simulink model "emulation"  (R2022b)
settings: Solver=FixedStepAuto  StartTime=0.0  StopTime=0.2  FixedStep=5e-8  RelTol=1e-3
libraries: spsVoltageMeasurementLib x5, fl_lib x4, spsParallelRLCBranchLib x4, spsACVoltageSourceLib x3, spsSecondOrderFilterLib x1, ee_lib x1, spspowerguiLib x1
settings Model: Creator=Motimon  LastModifiedBy=HP
settings ModelReferenceCC: EnableRefExpFcnMdlSchedulingChecks=on

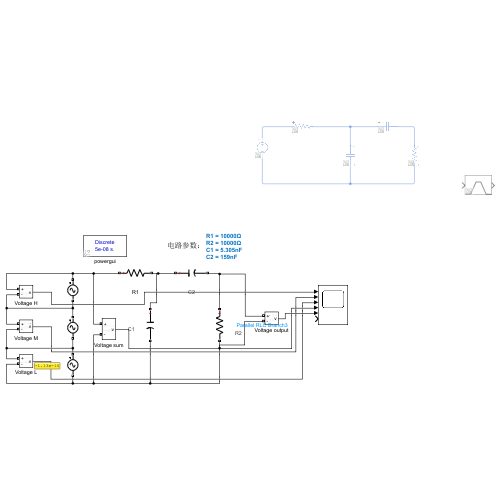
[thumbnail: Simulink's stored preview of the top-level diagram]
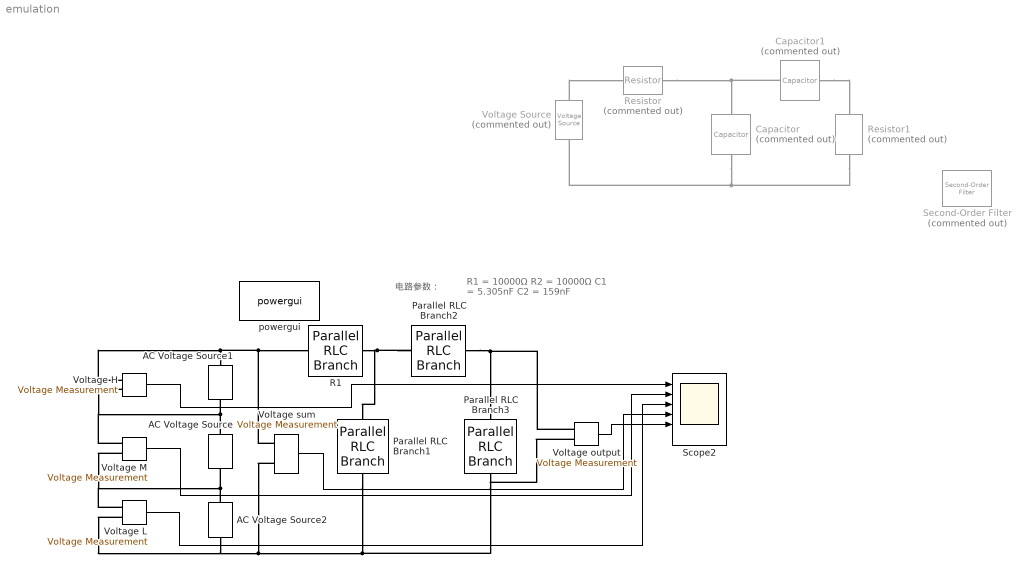
== system emulation ==
  note: 电路参数：
  note: R1 = 10000Ω
      | R2 = 10000Ω
      | C1 = 5.305nF
      | C2 = 159nF
  AC Voltage Source : spsACVoltageSourceLib/AC Voltage Source  Amplitude=0.5  Phase=0  Frequency=1550  SampleTime=0  Measurements=Voltage  BusType=swing  Pref=10e3  Qref=0  Qmin=-inf  Qmax=+inf
  AC Voltage Source1 : spsACVoltageSourceLib/AC Voltage Source  Amplitude=0.5  Phase=0  Frequency=60000  SampleTime=0  Measurements=Voltage  BusType=swing  Pref=10e3  Qref=0  Qmin=-inf  Qmax=+inf
  AC Voltage Source2 : spsACVoltageSourceLib/AC Voltage Source  Amplitude=0.5  Phase=0  Frequency=10  SampleTime=0  Measurements=Voltage  BusType=swing  Pref=10e3  Qref=0  Qmin=-inf  Qmax=+inf
  Capacitor : fl_lib/Electrical/Electrical Elements/Capacitor  Commented=on  c=1e-6 F  r=1e-6 Ohm  g=0 1/Ohm  i_specify=off  i_priority=None  i=0 A  i_nominal_specify=off  i_nominal_unit=A  i_nominal_value=1  v_specify=off  v_priority=None  v=0 V  v_nominal_specify=off  v_nominal_unit=V  v_nominal_value=1  vc_specify=off  vc_priority=High  vc=0 V  vc_nominal_specify=off  vc_nominal_unit=V  vc_nominal_value=1
  Capacitor1 : fl_lib/Electrical/Electrical Elements/Capacitor  Commented=on  c=1e-6 F  r=1e-6 Ohm  g=0 1/Ohm  i_specify=off  i_priority=None  i=0 A  i_nominal_specify=off  i_nominal_unit=A  i_nominal_value=1  v_specify=off  v_priority=None  v=0 V  v_nominal_specify=off  v_nominal_unit=V  v_nominal_value=1  vc_specify=off  vc_priority=High  vc=0 V  vc_nominal_specify=off  vc_nominal_unit=V  vc_nominal_value=1
  Parallel RLC Branch1 : spsParallelRLCBranchLib/Parallel RLC Branch  LConnTagsString=a  RConnTagsString=__new0  BranchType=C  Resistance=1  Inductance=1e-3  SetiL0=off  InitialCurrent=0  Capacitance=5.305e-9  Setx0=off  InitialVoltage=0  Measurements=None
      settings: AttributesFormatString=C1\n
  Parallel RLC Branch2 : spsParallelRLCBranchLib/Parallel RLC Branch  LConnTagsString=a  RConnTagsString=__new0  BranchType=C  Resistance=1  Inductance=1e-3  SetiL0=off  InitialCurrent=0  Capacitance=159e-9  Setx0=off  InitialVoltage=0  Measurements=None
      settings: AttributesFormatString=C2\n
  Parallel RLC Branch3 : spsParallelRLCBranchLib/Parallel RLC Branch  LConnTagsString=a  RConnTagsString=__new0  BranchType=R  Resistance=10000  Inductance=1e-3  SetiL0=off  InitialCurrent=0  Capacitance=1e-6  Setx0=off  InitialVoltage=0  Measurements=None
      settings: AttributesFormatString=R2\n
  R1 : spsParallelRLCBranchLib/Parallel RLC Branch  LConnTagsString=a  RConnTagsString=__new0  BranchType=R  Resistance=10000  Inductance=1e-3  SetiL0=off  InitialCurrent=0  Capacitance=1e-6  Setx0=off  InitialVoltage=0  Measurements=None
  Resistor : fl_lib/Electrical/Electrical Elements/Resistor  Commented=on  R=1 Ohm  i_specify=off  i_priority=None  i=0 A  i_nominal_specify=off  i_nominal_unit=A  i_nominal_value=1  v_specify=off  v_priority=None  v=0 V  v_nominal_specify=off  v_nominal_unit=V  v_nominal_value=1
  Resistor1 : fl_lib/Electrical/Electrical Elements/Resistor  Commented=on  R=1 Ohm  i_specify=off  i_priority=None  i=0 A  i_nominal_specify=off  i_nominal_unit=A  i_nominal_value=1  v_specify=off  v_priority=None  v=0 V  v_nominal_specify=off  v_nominal_unit=V  v_nominal_value=1
  Scope2 : Scope  NumInputPorts=6
  Second-Order Filter : spsSecondOrderFilterLib/Second-Order Filter  Commented=on  FilterType=Bandpass  Fo=547.723  Zeta=0.707  Ts=0  Initialize=on  Vac_Init="[1,  0,  100]"  Vdc_Init=0  PlotResponse=off  FreqRange=[0, 10000, 1]
  Voltage H : spsVoltageMeasurementLib/Voltage Measurement  PhasorSimulation=off  OutputType=Complex  PSBequivalent=0
  Voltage L : spsVoltageMeasurementLib/Voltage Measurement  PhasorSimulation=off  OutputType=Complex  PSBequivalent=0
  Voltage M : spsVoltageMeasurementLib/Voltage Measurement  PhasorSimulation=off  OutputType=Complex  PSBequivalent=0
  Voltage Source : ee_lib/Sources/Voltage Source  Commented=on  dc_voltage=0 V  ac_voltage=0 V  ac_shift=0 rad  ac_frequency=60 Hz  noise_mode=0  PSD=0 V^2/Hz  sample_time=1e-3 s  repeatability=1  user_seed=0  auto_seed=3499211588  i_specify=off  i_priority=None  i=0 A  i_nominal_specify=off  i_nominal_unit=A  i_nominal_value=1  v_specify=off  v_priority=None  v=0 V  v_nominal_specify=off  v_nominal_unit=V  v_nominal_value=1
  Voltage output : spsVoltageMeasurementLib/Voltage Measurement  PhasorSimulation=off  OutputType=Complex  PSBequivalent=0
  Voltage sum : spsVoltageMeasurementLib/Voltage Measurement  PhasorSimulation=off  OutputType=Complex  PSBequivalent=0
  powergui : spspowerguiLib/powergui  Priority=1  SimulationMode=Discrete  SampleTime=50e-9  frequency=60  Iterations=50  frequencyindice=1550  Pbase=100e6  ErrMax=1e-4  UnitsV=kV  UnitsW=MW  buscounter=0  FunctionMessages=off  echomessages=off  EnableUseOfTLC=off  CurrentSourceSwitches=off  DisableSnubberDevices=off  DisableRonSwitches=off  DisableVfSwitches=off  DisplayEquations=off  AutomaticDiscreteSolvers=off  SolverType=Tustin/Backward Euler (TBE)  Interpol=off  ExternalGateDelay=off  methode=off  Ts=100  x0status=blocks  SPID=on  SwTol=0  HookPort=off  NonlinearTolerance=1e-4  nMaxIteration=100  ContinueOnMaxIteration=off  RestoreLinks=warning  ResistiveCurrentMeasurement=off  Frange=[0:2:500]  Ylog=off  Xlog=on  ShowGrid=off  save=off  variable=ZData  structure=0  ZoomFFT=off  StartTime=0.0  cycles=1  DisplayStyle=1  fundamental=60  FreqAxis=off  MaxFrequency=1000  frequencyindicesteady=1  RmsSteady=1  display=off
  wires:
  Voltage L/1 -> Scope2/3
  Voltage M/1 -> Scope2/2
  Voltage H/1 -> Scope2/1
  Voltage sum/1 -> Scope2/4
  Voltage output/1 -> Scope2/5
  connections:
  Resistor/RConn1 -- Capacitor1/LConn1 -- Capacitor/LConn1
  Capacitor1/RConn1 -- Resistor1/LConn1
  Voltage Source/LConn1 -- Resistor/LConn1
  Capacitor/RConn1 -- Resistor1/RConn1 -- Voltage Source/RConn1
  R1/RConn1 -- Parallel RLC Branch2/LConn1 -- Parallel RLC Branch1/LConn1
  Parallel RLC Branch1/RConn1 -- Parallel RLC Branch3/RConn1 -- Voltage output/LConn2 -- Voltage L/LConn2 -- AC Voltage Source2/LConn1 -- Voltage sum/LConn2
  Parallel RLC Branch2/RConn1 -- Voltage output/LConn1 -- Parallel RLC Branch3/LConn1
  Voltage sum/LConn1 -- R1/LConn1 -- Voltage H/LConn1 -- AC Voltage Source1/RConn1
  AC Voltage Source/RConn1 -- Voltage H/LConn2 -- Voltage M/LConn1 -- AC Voltage Source1/LConn1
  AC Voltage Source2/RConn1 -- Voltage L/LConn1 -- Voltage M/LConn2 -- AC Voltage Source/LConn1
